simulink model "model6_1"  (R2025a)
settings: Solver=VariableStepAuto  StartTime=0.0  StopTime=10  RelTol=1e-3
values from neighbouring files (symbols this model uses):
  Tf = 1    [domaci6_1.m]
  Ts = 0.0001    [domaci6_1.m]
settings Model: Creator=neso  LastModifiedBy=Nenad

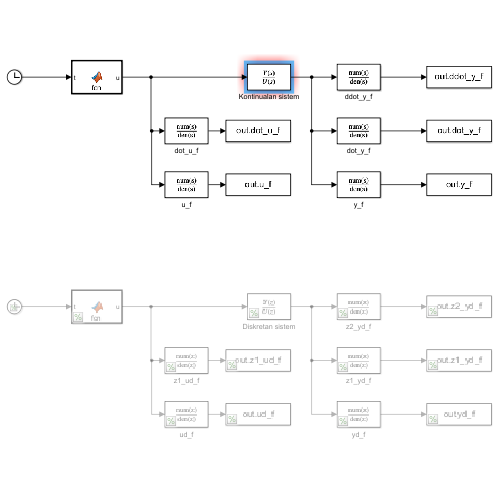
[thumbnail: Simulink's stored preview of the top-level diagram]
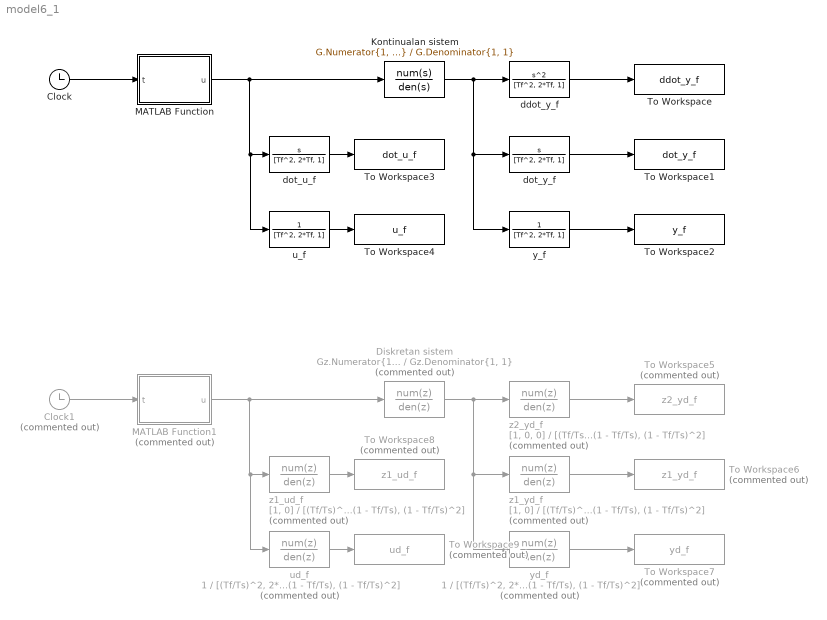
== system model6_1 ==
  Clock : Clock
  Clock1 : Clock  Commented=on
  Diskretan sistem : DiscreteTransferFcn  Commented=on  Numerator=Gz.Numerator{1, 1}  Denominator=Gz.Denominator{1, 1}
  Kontinualan sistem : TransferFcn  Numerator=G.Numerator{1, 1}  Denominator=G.Denominator{1, 1}
  MATLAB Function : MATLAB Function  TreatAsAtomicUnit=on
  MATLAB Function1 : MATLAB Function  Commented=on  TreatAsAtomicUnit=on
  To Workspace : ToWorkspace  VariableName=ddot_y_f  SaveFormat=Timeseries  SampleTime=-1
  To Workspace1 : ToWorkspace  VariableName=dot_y_f  SaveFormat=Timeseries  SampleTime=-1
  To Workspace2 : ToWorkspace  VariableName=y_f  SaveFormat=Timeseries  SampleTime=-1
  To Workspace3 : ToWorkspace  VariableName=dot_u_f  SaveFormat=Timeseries  SampleTime=-1
  To Workspace4 : ToWorkspace  VariableName=u_f  SaveFormat=Timeseries  SampleTime=-1
  To Workspace5 : ToWorkspace  Commented=on  VariableName=z2_yd_f  SaveFormat=Timeseries  SampleTime=-1
  To Workspace6 : ToWorkspace  Commented=on  VariableName=z1_yd_f  SaveFormat=Timeseries  SampleTime=-1
  To Workspace7 : ToWorkspace  Commented=on  VariableName=yd_f  SaveFormat=Timeseries  SampleTime=-1
  To Workspace8 : ToWorkspace  Commented=on  VariableName=z1_ud_f  SaveFormat=Timeseries  SampleTime=-1
  To Workspace9 : ToWorkspace  Commented=on  VariableName=ud_f  SaveFormat=Timeseries  SampleTime=-1
  ddot_y_f : TransferFcn  Numerator=[1, 0, 0]  Denominator=[Tf^2, 2*Tf, 1]
  dot_u_f : TransferFcn  Numerator=[1, 0]  Denominator=[Tf^2, 2*Tf, 1]
  dot_y_f : TransferFcn  Numerator=[1, 0]  Denominator=[Tf^2, 2*Tf, 1]
  u_f : TransferFcn  Numerator=1  Denominator=[Tf^2, 2*Tf, 1]
  ud_f : DiscreteTransferFcn  Commented=on  Numerator=1  Denominator=[(Tf/Ts)^2, 2*(Tf/Ts)*(1 - Tf/Ts), (1 - Tf/Ts)^2]
  y_f : TransferFcn  Numerator=1  Denominator=[Tf^2, 2*Tf, 1]
  yd_f : DiscreteTransferFcn  Commented=on  Numerator=1  Denominator=[(Tf/Ts)^2, 2*(Tf/Ts)*(1 - Tf/Ts), (1 - Tf/Ts)^2]
  z1_ud_f : DiscreteTransferFcn  Commented=on  Numerator=[1, 0]  Denominator=[(Tf/Ts)^2, 2*(Tf/Ts)*(1 - Tf/Ts), (1 - Tf/Ts)^2]
  z1_yd_f : DiscreteTransferFcn  Commented=on  Numerator=[1, 0]  Denominator=[(Tf/Ts)^2, 2*(Tf/Ts)*(1 - Tf/Ts), (1 - Tf/Ts)^2]
  z2_yd_f : DiscreteTransferFcn  Commented=on  Numerator=[1, 0, 0]  Denominator=[(Tf/Ts)^2, 2*(Tf/Ts)*(1 - Tf/Ts), (1 - Tf/Ts)^2]
  wires:
  MATLAB Function/1(u) -> u_f/1, dot_u_f/1, Kontinualan sistem/1
  Clock/1 -> MATLAB Function/1(t)
  Kontinualan sistem/1 -> y_f/1, dot_y_f/1, ddot_y_f/1
  ddot_y_f/1 -> To Workspace/1
  dot_y_f/1 -> To Workspace1/1
  y_f/1 -> To Workspace2/1
  dot_u_f/1 -> To Workspace3/1
  u_f/1 -> To Workspace4/1
  ud_f/1 -> To Workspace9/1
  Clock1/1 -> MATLAB Function1/1(t)
  z1_ud_f/1 -> To Workspace8/1
  MATLAB Function1/1(u) -> Diskretan sistem/1, ud_f/1, z1_ud_f/1
  Diskretan sistem/1 -> z2_yd_f/1, yd_f/1, z1_yd_f/1
  yd_f/1 -> To Workspace7/1
  z1_yd_f/1 -> To Workspace6/1
  z2_yd_f/1 -> To Workspace5/1

== matlab function model6_1/MATLAB Function ==
  data: t input; u output
function u = fcn(t)
    u = 0;
    fmax = 10;
    for i = 1:fmax
        u = u + sin(2 * pi * i * t);
    end

== matlab function model6_1/MATLAB Function1 ==
  data: t input; u output
function u = fcn(t)
    u = 0;
    fmax = 10;
    for i = 1:fmax
        u = u + sin(2 * pi * i * t);
    end
